simulink model "CollaborativeErgonomyControl"  (R2021b)
settings: Solver=FixedStepAuto  StartTime=0.0  StopTime=Config.SIMULATION_TIME  FixedStep=Config.tStep  RelTol=1e-3
InitFcn:
  | %% initialize the simulation
  | cd(fileparts(which(bdroot)));
  | initCollaborativeErgonomyControl;
StopFcn:
  | %% stop the simulation
  | cd(fileparts(which(bdroot)));
  | stopCollaborativeErgonomyControl;
values from neighbouring files (symbols this model uses):
  ConfigRobot1 = ConfigRobot    [initCollaborativeErgonomyControl.m]
  ConfigRobot2 = ConfigRobot    [initCollaborativeErgonomyControl.m]
undefined symbols (not defined in the file or in its folder): Config, ConfigObject
libraries: RobotStateLibrary x61, WBToolboxLibrary x40, MultiBodyLibrary x4, simulink x3
(part 2 of 2)

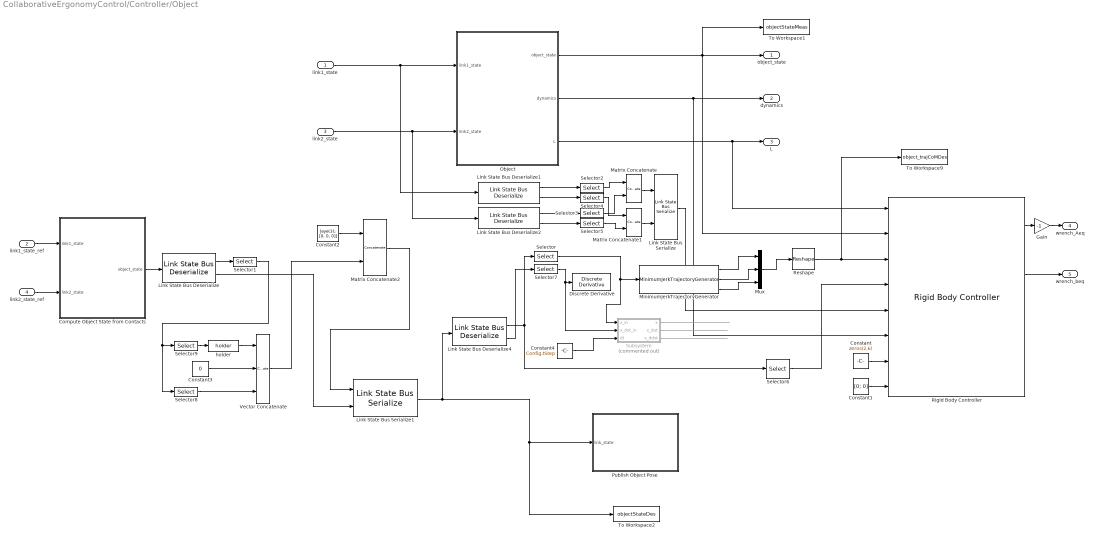
== system CollaborativeErgonomyControl/Controller/Object ==
  link1_state : Inport
  link1_state_ref : Inport  Port=2
  link2_state : Inport  Port=3
  link2_state_ref : Inport  Port=4
  Compute Object State from Contacts : Subsystem  AncestorBlock=MultiBodyLibrary/Compute Object State from Contacts
  Constant : Constant  Value=zeros(2,6)
  Constant1 : Constant  Value=[0; 0]
  Constant2 : Constant  Value=[eye(3); [0, 0, 0]]
  Constant3 : Constant  Value=0
  Constant4 : Constant  Value=Config.tStep
  Discrete Derivative : simulink/Discrete/Discrete Derivative  gainval=1.0  ICPrevScaledInput=0.0  OutMin=[]  OutMax=[]  OutDataType=fixdt(1, 16)  OutScaling=2^-10  DoSatur=off
  Gain : Gain  Gain=-1
  Link State Bus Deserialize{,1..2,4} (4 alike) : RobotStateLibrary/Link State Bus Deserialize  SystemSampleTime=-1  VariantActivationTime=update diagram  Latency=0  AutoFrameSizeCalculation=off
      settings: SourceProductName=robot-state-library
  Link State Bus Serialize : RobotStateLibrary/Link State Bus Serialize  SystemSampleTime=-1  VariantActivationTime=update diagram  Latency=0  AutoFrameSizeCalculation=off
      settings: SourceProductName=robot-state-library
  Link State Bus Serialize1 : RobotStateLibrary/Link State Bus Serialize  SystemSampleTime=-1  VariantActivationTime=update diagram  Latency=0  AutoFrameSizeCalculation=off
      settings: SourceProductName=robot-state-library
  Matrix Concatenate : Concatenate  Mode=Multidimensional array
  Matrix Concatenate1 : Concatenate  Mode=Multidimensional array
  Matrix Concatenate2 : Concatenate  Mode=Multidimensional array  ConcatenateDimension=2
  MinimumJerkTrajectoryGenerator : WBToolboxLibrary/Utilities/MinimumJerkTrajectoryGenerator  externalSettlingTime=off  settlingTime=3  sampleTime=0.01  resetOnSettlingTime=off  firstDerivatives=on  secondDerivatives=on  explicitInitialValue=off
      settings: SourceProductName=WholeBodyToolbox
  Mux : Mux  Inputs=3
  Object : Subsystem
  Publish Object Pose : Subsystem
  Reshape : Reshape  OutputDimensionality=Customize  OutputDimensions=[3,3]
  Rigid Body Controller : MultiBodyLibrary/Rigid Body Controller  GainMomentum=ConfigObject.Gains.GainMomentum  linksUseConstraintMatrix=ConfigObject.linksUseConstraintMatrix
      settings: SourceProductName=multi-body-library
  Selector : Selector  NumberOfDimensions=2  InputPortWidth=3  IndexOptions=Index vector (dialog),Index vector (dialog)  Indices=[1 2 3],4  OutputSizes=1,1
  Selector1 : Selector  NumberOfDimensions=2  InputPortWidth=3  IndexOptions=Index vector (dialog),Index vector (dialog)  Indices=[1 2 3 4],4  OutputSizes=1,1
  Selector2 : Selector  NumberOfDimensions=2  InputPortWidth=3  IndexOptions=Starting index (dialog),Index vector (dialog)  Indices=9,[1 2 3 4]  OutputSizes=8,1
  Selector3 : Selector  NumberOfDimensions=2  InputPortWidth=3  IndexOptions=Starting index (dialog),Index vector (dialog)  Indices=9,[1 2 3 4]  OutputSizes=8,1
  Selector4 : Selector  NumberOfDimensions=2  InputPortWidth=3  IndexOptions=Starting index (dialog),Index vector (dialog)  Indices=13,1  OutputSizes=12,1
  Selector5 : Selector  NumberOfDimensions=2  InputPortWidth=3  IndexOptions=Starting index (dialog),Index vector (dialog)  Indices=13,1  OutputSizes=12,1
  Selector6 : Selector  NumberOfDimensions=2  InputPortWidth=3  IndexOptions=Index vector (dialog),Index vector (dialog)  Indices=[1 2 3],[1 2 3]  OutputSizes=1,1
  Selector7 : Selector  IndexOptions=Index vector (dialog)  Indices=[1 2 3]  OutputSizes=1
  Selector8 : Selector  IndexOptions=Index vector (dialog)  Indices=[3 4]  OutputSizes=1
  Selector9 : Selector  IndexOptions=Index vector (dialog)  Indices=[1]  OutputSizes=1
  Subsystem : Subsystem  Commented=on
  To Workspace1 : ToWorkspace  VariableName=objectStateMeas  SaveFormat=Timeseries  SampleTime=-1
  To Workspace2 : ToWorkspace  VariableName=objectStateDes  SaveFormat=Timeseries  SampleTime=-1
  To Workspace9 : ToWorkspace  VariableName=object_trajCoMDes  SaveFormat=Timeseries  SampleTime=-1
  Vector Concatenate : Concatenate  NumInputs=3
  "holder " : WBToolboxLibrary/Utilities/holder 
      settings: SourceProductName=WholeBodyToolbox
  object_state : Outport
  dynamics : Outport  Port=2
  L : Outport  Port=3
  wrench_Aeq : Outport  Port=4
  wrench_beq : Outport  Port=5
  wires:
  Object/3(L) -> Rigid Body Controller/1, L/1
  link2_state_ref/1 -> Compute Object State from Contacts/2(link2_state)
  link2_state/1 -> Link State Bus Deserialize2/1, Object/2(link2_state)
  Object/1(object_state) -> To Workspace1/1, Rigid Body Controller/2, object_state/1
  Object/2(dynamics) -> Rigid Body Controller/6, dynamics/1
  link1_state_ref/1 -> Compute Object State from Contacts/1(link1_state)
  Compute Object State from Contacts/1(object_state) -> Link State Bus Deserialize/1
  Mux/1 -> Reshape/1
  Reshape/1 -> To Workspace9/1, Rigid Body Controller/3
  link1_state/1 -> Link State Bus Deserialize1/1, Object/1(link1_state)
  Link State Bus Deserialize1/1 -> Selector2/1
  Link State Bus Deserialize2/1 -> Selector3/1
  Selector2/1 -> Matrix Concatenate/1
  Selector3/1 -> Matrix Concatenate/2
  Link State Bus Deserialize1/2 -> Selector4/1
  Link State Bus Deserialize2/2 -> Selector5/1
  Selector5/1 -> Matrix Concatenate1/2
  Selector4/1 -> Matrix Concatenate1/1
  Matrix Concatenate/1 -> Link State Bus Serialize/1
  Matrix Concatenate1/1 -> Link State Bus Serialize/2
  Rigid Body Controller/1 -> Gain/1
  Rigid Body Controller/2 -> wrench_beq/1
  Gain/1 -> wrench_Aeq/1
  Constant1/1 -> Rigid Body Controller/8
  Constant/1 -> Rigid Body Controller/7
  Link State Bus Serialize/1 -> Rigid Body Controller/5
  Selector7/1 -> Subsystem/2(x_dot_in), Discrete Derivative/1
  Selector/1 -> Subsystem/1(x_in), MinimumJerkTrajectoryGenerator/1
  Selector6/1 -> Rigid Body Controller/4
  Link State Bus Deserialize/2 -> Link State Bus Serialize1/2
  Link State Bus Deserialize/1 -> Selector1/1
  Constant2/1 -> Matrix Concatenate2/1
  Matrix Concatenate2/1 -> Link State Bus Serialize1/1
  Link State Bus Serialize1/1 -> Link State Bus Deserialize4/1, To Workspace2/1, Publish Object Pose/1(link_state)
  Link State Bus Deserialize4/1 -> Selector/1, Selector6/1
  Link State Bus Deserialize4/2 -> Selector7/1
  Vector Concatenate/1 -> Matrix Concatenate2/2
  Constant3/1 -> Vector Concatenate/2
  Selector8/1 -> Vector Concatenate/3
  Selector9/1 -> "holder "/1
  "holder "/1 -> Vector Concatenate/1
  Selector1/1 -> Selector8/1, Selector9/1
  Constant4/1 -> Subsystem/3(dt)
  Subsystem/1(x) -> ?
  Subsystem/2(x_dot) -> ?
  Subsystem/3(x_ddot) -> ?
  MinimumJerkTrajectoryGenerator/1 -> Mux/1
  MinimumJerkTrajectoryGenerator/2 -> Mux/2
  MinimumJerkTrajectoryGenerator/3 -> Mux/3

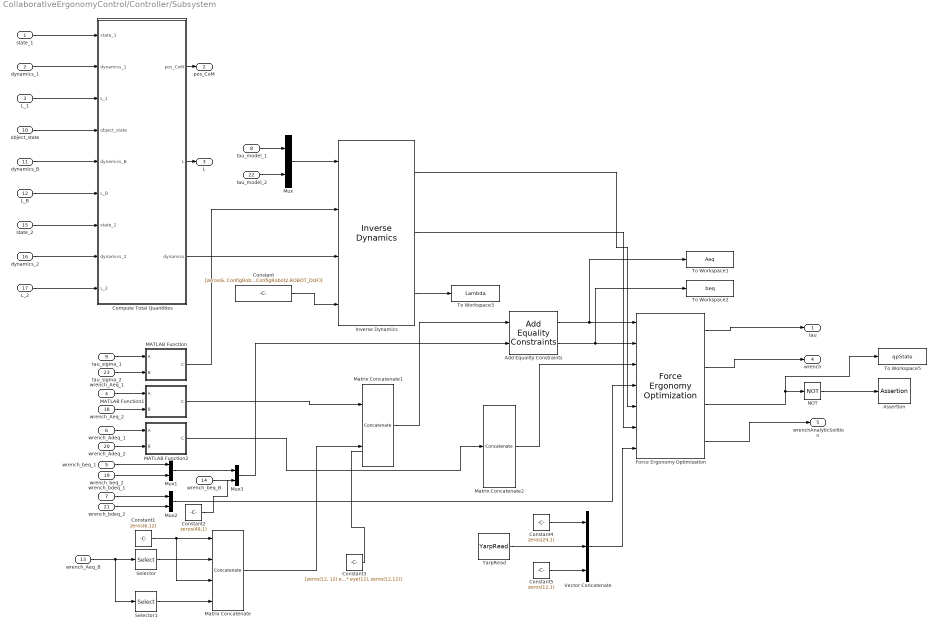
== system CollaborativeErgonomyControl/Controller/Subsystem ==
  state_1 : Inport
  dynamics_1 : Inport  Port=2
  L_1 : Inport  Port=3
  wrench_Aeq_1 : Inport  Port=4
  wrench_beq_1 : Inport  Port=5
  wrench_Adeq_1 : Inport  Port=6
  wrench_bdeq_1 : Inport  Port=7
  tau_model_1 : Inport  Port=8
  tau_sigma_1 : Inport  Port=9
  object_state : Inport  Port=10
  dynamics_B : Inport  Port=11
  L_B : Inport  Port=12
  wrench_Aeq_B : Inport  Port=13
  wrench_beq_B : Inport  Port=14
  state_2 : Inport  Port=15
  dynamics_2 : Inport  Port=16
  L_2 : Inport  Port=17
  wrench_Aeq_2 : Inport  Port=18
  wrench_beq_2 : Inport  Port=19
  wrench_Adeq_2 : Inport  Port=20
  wrench_bdeq_2 : Inport  Port=21
  tau_model_2 : Inport  Port=22
  tau_sigma_2 : Inport  Port=23
  Add Equality Constraints : RobotStateLibrary/Add Equality Constraints  Aeq_add=Config.wrench_Aeq_const  beq_add=Config.wrench_beq_const
      settings: SourceProductName=robot-state-library
  Assertion : Assertion
  Compute Total Quantities : Subsystem
  Constant : Constant  Value=[zeros(6, ConfigRobot1.ROBOT_DOF + ConfigRobot2.ROBOT_DOF); [eye(ConfigRobot1.ROBOT_DOF), zeros(ConfigRobot1.ROBOT_DOF, ConfigRobot2.ROBOT_DOF)]; zeros(6, ConfigRobot1.ROBOT_DOF + ConfigRobot2.ROBOT_DOF); [zeros(ConfigRobot2.ROBOT_DOF, ConfigRobot1.ROBOT_DOF), eye(ConfigRobot2.ROBOT_DOF)]; zeros(6, ConfigRobot1.ROBOT_DOF + ConfigRobot2.ROBOT_DOF)]
  Constant1 : Constant  Value=zeros(6,12)
  Constant2 : Constant  Value=zeros(48,1)
  Constant3 : Constant  Value=[zeros(12, 12) eye(12) zeros(12, 24); zeros(12, 24) zeros(12, 12) eye(12); 0.01 * eye(12) zeros(12,36); zeros(12,24) 0.01 * eye(12), zeros(12,12)]
  Constant4 : Constant  Value=zeros(24,1)
  Constant5 : Constant  Value=zeros(12,1)
  Force Ergonomy Optimization : RobotStateLibrary/Force Ergonomy Optimization  InvTol=Config.Reg.AInvTol  regularizationHessian=Config.Reg.Hessian  minimizationWeight=Config.Gains.tauMinimization  regularizationYDes=Config.Reg.DesWrenchReg
      settings: SourceProductName=robot-state-library
  Inverse Dynamics : RobotStateLibrary/Inverse Dynamics  Reg=Config.Reg  fixedLinkVelcityComponents=Config.fixedLinkVelcityComponents
      settings: SourceProductName=robot-state-library
  MATLAB Function : MATLAB Function  TreatAsAtomicUnit=on
  MATLAB Function1 : MATLAB Function  TreatAsAtomicUnit=on
  MATLAB Function2 : MATLAB Function  TreatAsAtomicUnit=on
  Matrix Concatenate : Concatenate  NumInputs=4  Mode=Multidimensional array  ConcatenateDimension=2
  Matrix Concatenate1 : Concatenate  Mode=Multidimensional array
  Matrix Concatenate2 : Concatenate  NumInputs=1  Mode=Multidimensional array
  Mux{,1..3} (4 alike) : Mux  Inputs=2
  NOT : Logic  Operator=NOT  IconShape=distinctive  AllPortsSameDT=off  OutDataTypeStr=boolean
  Selector : Selector  NumberOfDimensions=2  InputPortWidth=3  IndexOptions=Starting index (dialog),Starting index (dialog)  Indices=1,1  OutputSizes=6,12
  Selector1 : Selector  NumberOfDimensions=2  InputPortWidth=3  IndexOptions=Starting index (dialog),Starting index (dialog)  Indices=1,13  OutputSizes=6,12
  To Workspace1 : ToWorkspace  VariableName=Aeq  SaveFormat=Timeseries  SampleTime=-1
  To Workspace2 : ToWorkspace  VariableName=beq  SaveFormat=Timeseries  SampleTime=-1
  To Workspace3 : ToWorkspace  VariableName=Lambda  SaveFormat=Timeseries  SampleTime=-1
  To Workspace5 : ToWorkspace  VariableName=qpState  SaveFormat=Timeseries  SampleTime=-1
  Vector Concatenate : Concatenate  NumInputs=3
  YarpRead : WBToolboxLibrary/Utilities/YarpRead  portName=ConfigRobot2.Ports.WRENCH_FEET  signalSize=12  timeout=0.5  blocking=off  timestamp=off  autoconnect=on  errorOnConnection=on
      settings: SourceProductName=WholeBodyToolbox
  tau : Outport
  pos_CoM : Outport  Port=2
  L : Outport  Port=3
  wrench : Outport  Port=4
  wrenchAnalyticSolition : Outport  Port=5
  wires:
  wrench_Aeq_2/1 -> MATLAB Function1/2(B)
  Mux/1 -> Inverse Dynamics/1
  Compute Total Quantities/2(L) -> L/1
  Force Ergonomy Optimization/1 -> tau/1
  wrench_bdeq_1/1 -> Mux2/1
  Selector/1 -> Matrix Concatenate/2
  wrench_bdeq_2/1 -> Mux2/2
  state_2/1 -> Compute Total Quantities/7(state_2)
  dynamics_2/1 -> Compute Total Quantities/8(dynamics_2)
  dynamics_1/1 -> Compute Total Quantities/2(dynamics_1)
  tau_sigma_1/1 -> MATLAB Function/1(A)
  dynamics_B/1 -> Compute Total Quantities/5(dynamics_B)
  wrench_Adeq_2/1 -> MATLAB Function2/2(B)
  Compute Total Quantities/3(dynamics) -> Inverse Dynamics/3
  Mux2/1 -> Force Ergonomy Optimization/4
  object_state/1 -> Compute Total Quantities/4(object_state)
  MATLAB Function/1(C) -> Inverse Dynamics/2
  L_1/1 -> Compute Total Quantities/3(L_1)
  wrench_Aeq_1/1 -> MATLAB Function1/1(A)
  Force Ergonomy Optimization/2 -> wrench/1
  Mux3/1 -> Add Equality Constraints/2
  Constant1/1 -> Matrix Concatenate/3, Matrix Concatenate/1
  Compute Total Quantities/1(pos_CoM) -> pos_CoM/1
  wrench_Aeq_B/1 -> Selector1/1, Selector/1
  tau_model_1/1 -> Mux/1
  state_1/1 -> Compute Total Quantities/1(state_1)
  wrench_beq_2/1 -> Mux1/2
  Mux1/1 -> Mux3/1
  Matrix Concatenate1/1 -> Add Equality Constraints/1
  wrench_beq_B/1 -> Mux3/2
  Matrix Concatenate/1 -> Matrix Concatenate1/2
  MATLAB Function1/1(C) -> Matrix Concatenate1/1
  wrench_beq_1/1 -> Mux1/1
  Inverse Dynamics/1 -> Force Ergonomy Optimization/5
  tau_model_2/1 -> Mux/2
  L_B/1 -> Compute Total Quantities/6(L_B)
  Add Equality Constraints/2 -> To Workspace2/1, Force Ergonomy Optimization/2
  wrench_Adeq_1/1 -> MATLAB Function2/1(A)
  tau_sigma_2/1 -> MATLAB Function/2(B)
  L_2/1 -> Compute Total Quantities/9(L_2)
  Constant/1 -> Inverse Dynamics/4
  Inverse Dynamics/2 -> Force Ergonomy Optimization/6
  Selector1/1 -> Matrix Concatenate/4
  NOT/1 -> Assertion/1
  Force Ergonomy Optimization/3 -> To Workspace5/1, NOT/1
  Add Equality Constraints/1 -> To Workspace1/1, Force Ergonomy Optimization/1
  Force Ergonomy Optimization/4 -> wrenchAnalyticSolition/1
  Inverse Dynamics/3 -> To Workspace3/1
  MATLAB Function2/1(C) -> Matrix Concatenate2/1
  Matrix Concatenate2/1 -> Force Ergonomy Optimization/3
  Constant2/1 -> ?
  Constant3/1 -> ?
  Vector Concatenate/1 -> Force Ergonomy Optimization/7
  Constant4/1 -> Vector Concatenate/1
  YarpRead/1 -> Vector Concatenate/2
  Constant5/1 -> Vector Concatenate/3

== system CollaborativeErgonomyControl/Dump and visualize/Time Scope ==
  yarp_time : Inport
  simulink_time : Inport  Port=2
  Enable : EnablePort
  Difference : simulink/Discrete/Difference  ICPrevInput=0.0  OutMin=[]  OutMax=[]  OutDataType=fixdt(1, 16)  OutScaling=2^-10  DoSatur=off
  Difference1 : simulink/Discrete/Difference  ICPrevInput=0.0  OutMin=[]  OutMax=[]  OutDataType=fixdt(1, 16)  OutScaling=2^-10  DoSatur=off
  Minus : Sum  Inputs=-+
  Mux : Mux  Inputs=2
  Mux1 : Mux  Inputs=2
  Time Scope : Scope  NumInputPorts=2
  "holder " : WBToolboxLibrary/Utilities/holder 
      settings: SourceProductName=WholeBodyToolbox
  wires:
  yarp_time/1 -> "holder "/1, Minus/2, Difference/1  "time"
  "holder "/1 -> Minus/1
  simulink_time/1 -> Mux/2, Difference1/1  "simulink time"
  Minus/1 -> Mux/1  "yarp time"
  Mux/1 -> Time Scope/1
  Difference/1 -> Mux1/1  "yarp time step"
  Difference1/1 -> Mux1/2  "simulink time step"
  Mux1/1 -> Time Scope/2

== system CollaborativeErgonomyControl/synchronizer/GAZEBO_SYNCHRONIZER ==
  Enable : EnablePort
  Simulator Synchronizer : WBToolboxLibrary/Utilities/Simulator Synchronizer  period=Config.tStep  serverPortName='/clock/rpc'  clientPortName='/WBT_synchronizer/rpc:o'
      settings: SourceProductName=WholeBodyToolbox

== system CollaborativeErgonomyControl/synchronizer/REAL_TIME_SYNC ==
  Enable : EnablePort
  Real Time Synchronizer : WBToolboxLibrary/Utilities/Real Time Synchronizer  period=Config.tStep
      settings: SourceProductName=WholeBodyToolbox

== system CollaborativeErgonomyControl/Controller/Model 1/Initial State Holder ==
  state : Inport
  State Bus Deserializer : RobotStateLibrary/State Bus Deserializer  SystemSampleTime=-1  VariantActivationTime=update diagram  Latency=0  AutoFrameSizeCalculation=off
      settings: SourceProductName=robot-state-library
  State Bus Serializer : RobotStateLibrary/State Bus Serializer  SystemSampleTime=-1  VariantActivationTime=update diagram  Latency=0  AutoFrameSizeCalculation=off
      settings: SourceProductName=robot-state-library
  holder {,1..3} (4 alike) : WBToolboxLibrary/Utilities/holder 
      settings: SourceProductName=WholeBodyToolbox
  state0 : Outport
  wires:
  State Bus Deserializer/2 -> holder 1/1
  State Bus Deserializer/4 -> holder 3/1
  holder 1/1 -> State Bus Serializer/2
  holder 3/1 -> State Bus Serializer/4
  State Bus Deserializer/1 -> "holder "/1
  state/1 -> State Bus Deserializer/1
  holder 2/1 -> State Bus Serializer/3
  State Bus Serializer/1 -> state0/1
  "holder "/1 -> State Bus Serializer/1
  State Bus Deserializer/3 -> holder 2/1

== system CollaborativeErgonomyControl/Controller/Model 3/Initial State Holder ==
  state : Inport
  State Bus Deserializer : RobotStateLibrary/State Bus Deserializer  SystemSampleTime=-1  VariantActivationTime=update diagram  Latency=0  AutoFrameSizeCalculation=off
      settings: SourceProductName=robot-state-library
  State Bus Serializer : RobotStateLibrary/State Bus Serializer  SystemSampleTime=-1  VariantActivationTime=update diagram  Latency=0  AutoFrameSizeCalculation=off
      settings: SourceProductName=robot-state-library
  holder {,1..3} (4 alike) : WBToolboxLibrary/Utilities/holder 
      settings: SourceProductName=WholeBodyToolbox
  state0 : Outport
  wires:
  State Bus Deserializer/2 -> holder 1/1
  State Bus Deserializer/4 -> holder 3/1
  holder 1/1 -> State Bus Serializer/2
  holder 3/1 -> State Bus Serializer/4
  State Bus Deserializer/1 -> "holder "/1
  state/1 -> State Bus Deserializer/1
  holder 2/1 -> State Bus Serializer/3
  State Bus Serializer/1 -> state0/1
  "holder "/1 -> State Bus Serializer/1
  State Bus Deserializer/3 -> holder 2/1

== system CollaborativeErgonomyControl/Controller/Object/Compute Object State from Contacts ==
  link1_state : Inport
  link2_state : Inport  Port=2
  Compute Object Pose From Contacts : Subsystem
  Compute Object Velocity From Contacts : Subsystem
  Link State Bus Deserialize : RobotStateLibrary/Link State Bus Deserialize  SystemSampleTime=-1  VariantActivationTime=update diagram  Latency=0  AutoFrameSizeCalculation=off
      settings: SourceProductName=robot-state-library
  Link State Bus Deserialize1 : RobotStateLibrary/Link State Bus Deserialize  SystemSampleTime=-1  VariantActivationTime=update diagram  Latency=0  AutoFrameSizeCalculation=off
      settings: SourceProductName=robot-state-library
  Link State Bus Serialize : RobotStateLibrary/Link State Bus Serialize  SystemSampleTime=-1  VariantActivationTime=update diagram  Latency=0  AutoFrameSizeCalculation=off
      settings: SourceProductName=robot-state-library
  object_state : Outport
  wires:
  Link State Bus Serialize/1 -> object_state/1
  Compute Object Velocity From Contacts/1(v_b) -> Link State Bus Serialize/2
  link2_state/1 -> Link State Bus Deserialize1/1
  link1_state/1 -> Link State Bus Deserialize/1
  Compute Object Pose From Contacts/1(w_H_b) -> Compute Object Velocity From Contacts/5(w_H_B), Link State Bus Serialize/1
  Link State Bus Deserialize1/1 -> Compute Object Pose From Contacts/2(w_H_2), Compute Object Velocity From Contacts/4(w_H_2)
  Link State Bus Deserialize1/2 -> Compute Object Velocity From Contacts/2(v_2)
  Link State Bus Deserialize/2 -> Compute Object Velocity From Contacts/1(v_1)
  Link State Bus Deserialize/1 -> Compute Object Pose From Contacts/1(w_H_1), Compute Object Velocity From Contacts/3(w_H_1)

== system CollaborativeErgonomyControl/Controller/Object/Object ==
  link1_state : Inport
  link2_state : Inport  Port=2
  Constant : Constant  Value=ConfigObject.contacts
  Constant1 : Constant  Value=ConfigObject.MassMatrix
  Get Object State and Dynamics : MultiBodyLibrary/Get Object State and Dynamics  SystemSampleTime=-1  VariantActivationTime=update diagram  Latency=0  AutoFrameSizeCalculation=off
      settings: SourceProductName=multi-body-library
  Publish Object Pose : Subsystem
  object_state : Outport
  dynamics : Outport  Port=2
  L : Outport  Port=3
  wires:
  link1_state/1 -> Get Object State and Dynamics/1
  Get Object State and Dynamics/1 -> object_state/1, Publish Object Pose/1(link_state)
  Constant1/1 -> Get Object State and Dynamics/4
  link2_state/1 -> Get Object State and Dynamics/2
  Get Object State and Dynamics/2 -> dynamics/1
  Constant/1 -> Get Object State and Dynamics/3
  Get Object State and Dynamics/3 -> L/1

== system CollaborativeErgonomyControl/Controller/Object/Publish Object Pose ==
  link_state : Inport
  Link State Bus Deserialize : RobotStateLibrary/Link State Bus Deserialize  SystemSampleTime=-1  VariantActivationTime=update diagram  Latency=0  AutoFrameSizeCalculation=off
      settings: SourceProductName=robot-state-library
  Pose Yarp Publisher : RobotStateLibrary/Pose Yarp Publisher  portName='/collaborativeController/boxRef/basePose:o'
      settings: SourceProductName=robot-state-library
  wires:
  Link State Bus Deserialize/1 -> Pose Yarp Publisher/1
  link_state/1 -> Link State Bus Deserialize/1

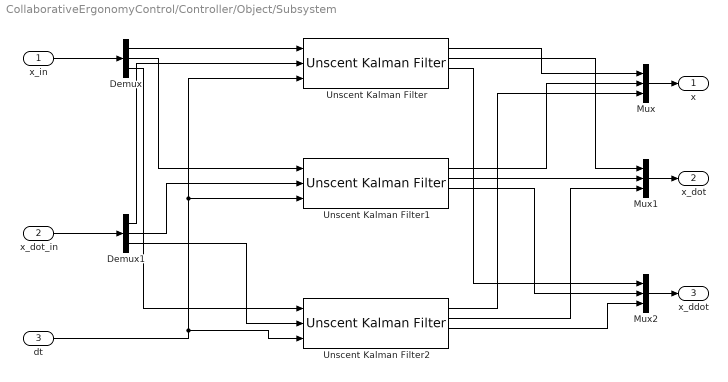
== system CollaborativeErgonomyControl/Controller/Object/Subsystem ==
  x_in : Inport
  x_dot_in : Inport  Port=2
  dt : Inport  Port=3
  Demux : Demux  Outputs=3
  Demux1 : Demux  Outputs=3
  Mux : Mux  Inputs=3
  Mux1 : Mux  Inputs=3
  Mux2 : Mux  Inputs=3
  Unscent Kalman Filter : RobotStateLibrary/Unscent Kalman Filter  SystemSampleTime=-1  VariantActivationTime=update diagram  Latency=0  AutoFrameSizeCalculation=off
      settings: SourceProductName=robot-state-library
  Unscent Kalman Filter1 : RobotStateLibrary/Unscent Kalman Filter  SystemSampleTime=-1  VariantActivationTime=update diagram  Latency=0  AutoFrameSizeCalculation=off
      settings: SourceProductName=robot-state-library
  Unscent Kalman Filter2 : RobotStateLibrary/Unscent Kalman Filter  SystemSampleTime=-1  VariantActivationTime=update diagram  Latency=0  AutoFrameSizeCalculation=off
      settings: SourceProductName=robot-state-library
  x : Outport
  x_dot : Outport  Port=2
  x_ddot : Outport  Port=3
  wires:
  x_in/1 -> Demux/1
  x_dot_in/1 -> Demux1/1
  dt/1 -> Unscent Kalman Filter2/3, Unscent Kalman Filter1/3, Unscent Kalman Filter/3
  Mux/1 -> x/1
  Mux1/1 -> x_dot/1
  Mux2/1 -> x_ddot/1
  Unscent Kalman Filter/1 -> Mux/1
  Unscent Kalman Filter1/1 -> Mux/2
  Unscent Kalman Filter2/1 -> Mux/3
  Unscent Kalman Filter/2 -> Mux1/1
  Unscent Kalman Filter1/2 -> Mux1/2
  Unscent Kalman Filter2/2 -> Mux1/3
  Unscent Kalman Filter/3 -> Mux2/1
  Unscent Kalman Filter1/3 -> Mux2/2
  Unscent Kalman Filter2/3 -> Mux2/3
  Demux/1 -> Unscent Kalman Filter/1
  Demux/2 -> Unscent Kalman Filter1/1
  Demux/3 -> Unscent Kalman Filter2/1
  Demux1/1 -> Unscent Kalman Filter/2
  Demux1/2 -> Unscent Kalman Filter1/2
  Demux1/3 -> Unscent Kalman Filter2/2

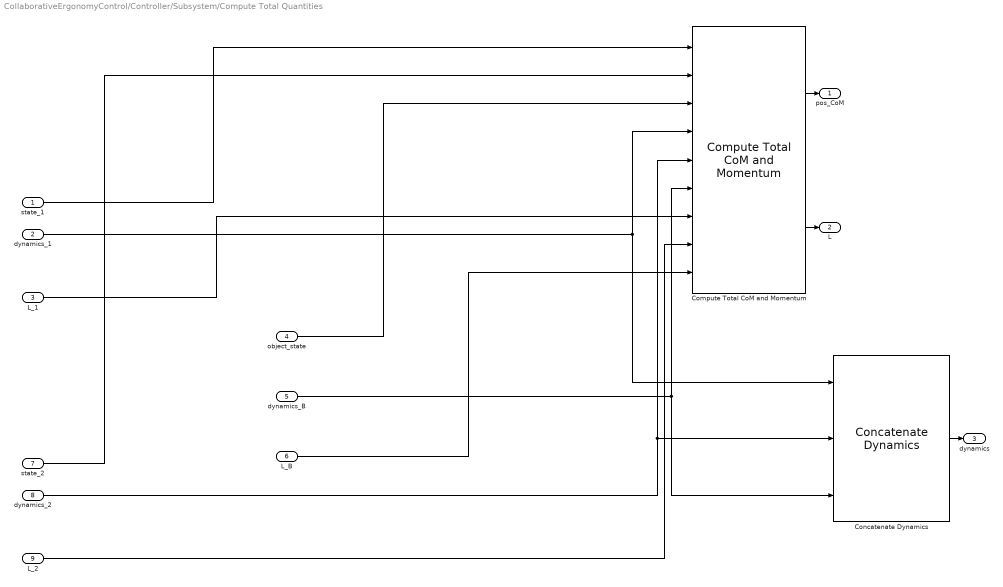
== system CollaborativeErgonomyControl/Controller/Subsystem/Compute Total Quantities ==
  state_1 : Inport
  dynamics_1 : Inport  Port=2
  L_1 : Inport  Port=3
  object_state : Inport  Port=4
  dynamics_B : Inport  Port=5
  L_B : Inport  Port=6
  state_2 : Inport  Port=7
  dynamics_2 : Inport  Port=8
  L_2 : Inport  Port=9
  Compute Total CoM and Momentum : MultiBodyLibrary/Compute Total CoM and Momentum  SystemSampleTime=-1  VariantActivationTime=update diagram  Latency=0  AutoFrameSizeCalculation=off
      settings: SourceProductName=multi-body-library
  Concatenate Dynamics : MultiBodyLibrary/Concatenate Dynamics  SystemSampleTime=-1  VariantActivationTime=update diagram  Latency=0  AutoFrameSizeCalculation=off
      settings: SourceProductName=multi-body-library
  pos_CoM : Outport
  L : Outport  Port=2
  dynamics : Outport  Port=3
  wires:
  L_2/1 -> Compute Total CoM and Momentum/8
  Compute Total CoM and Momentum/2 -> L/1
  L_B/1 -> Compute Total CoM and Momentum/9
  dynamics_2/1 -> Compute Total CoM and Momentum/5, Concatenate Dynamics/2
  Compute Total CoM and Momentum/1 -> pos_CoM/1
  dynamics_B/1 -> Compute Total CoM and Momentum/6, Concatenate Dynamics/3
  L_1/1 -> Compute Total CoM and Momentum/7
  object_state/1 -> Compute Total CoM and Momentum/3
  dynamics_1/1 -> Compute Total CoM and Momentum/4, Concatenate Dynamics/1
  Concatenate Dynamics/1 -> dynamics/1
  state_2/1 -> Compute Total CoM and Momentum/2
  state_1/1 -> Compute Total CoM and Momentum/1

== system CollaborativeErgonomyControl/Controller/Object/Compute Object State from Contacts/Compute Object Pose From Contacts ==
  w_H_1 : Inport
  w_H_2 : Inport  Port=2
  Compute Object pose from contacts : MATLAB Function  TreatAsAtomicUnit=on
  w_H_b : Outport
  wires:
  w_H_1/1 -> Compute Object pose from contacts/1(w_H_1)
  Compute Object pose from contacts/1(w_H_b) -> w_H_b/1
  w_H_2/1 -> Compute Object pose from contacts/2(w_H_2)

== system CollaborativeErgonomyControl/Controller/Object/Compute Object State from Contacts/Compute Object Velocity From Contacts ==
  v_1 : Inport
  v_2 : Inport  Port=2
  w_H_1 : Inport  Port=3
  w_H_2 : Inport  Port=4
  w_H_B : Inport  Port=5
  Compute Object velocity : MATLAB Function  TreatAsAtomicUnit=on
  v_b : Outport
  wires:
  Compute Object velocity/1(v_b) -> v_b/1
  v_2/1 -> Compute Object velocity/2(v_2)
  v_1/1 -> Compute Object velocity/1(v_1)
  w_H_B/1 -> Compute Object velocity/5(w_H_B)
  w_H_2/1 -> Compute Object velocity/4(w_H_2)
  w_H_1/1 -> Compute Object velocity/3(w_H_1)

== system CollaborativeErgonomyControl/Controller/Object/Object/Publish Object Pose ==
  link_state : Inport
  Link State Bus Deserialize : RobotStateLibrary/Link State Bus Deserialize  SystemSampleTime=-1  VariantActivationTime=update diagram  Latency=0  AutoFrameSizeCalculation=off
      settings: SourceProductName=robot-state-library
  Pose Yarp Publisher : RobotStateLibrary/Pose Yarp Publisher  portName='/collaborativeController/box/basePose:o'
      settings: SourceProductName=robot-state-library
  wires:
  Link State Bus Deserialize/1 -> Pose Yarp Publisher/1
  link_state/1 -> Link State Bus Deserialize/1

== matlab function CollaborativeErgonomyControl/Controller/Subsystem/MATLAB Function1 ==
  data: A input; C output; B input
function C = fcn(A, B)

C = blkdiag(A, B);

end

== matlab function CollaborativeErgonomyControl/Controller/Subsystem/MATLAB Function ==
  data: A input; C output; B input
function C = fcn(A, B)

C = blkdiag(A, B);

end

== matlab function CollaborativeErgonomyControl/Controller/Subsystem/MATLAB Function2 ==
  data: A input; C output; B input
function C = fcn(A, B)

C = blkdiag(A, B);

end

== matlab function CollaborativeErgonomyControl/Controller/Object/Compute Object State from Contacts/Compute Object Pose From Contacts/Compute Object pose from contacts ==
  data: w_H_1 input; w_H_b output; w_H_2 input
function w_H_b = computeObjectPoseFromContactsFCN(w_H_1, w_H_2)

w_H_b = mbl.computeObjectPoseFromContacts(w_H_1, w_H_2, true, true);

end

== matlab function CollaborativeErgonomyControl/Controller/Object/Compute Object State from Contacts/Compute Object Velocity From Contacts/Compute Object velocity ==
  data: v_1 input; v_b output; v_2 input; w_H_1 input; w_H_2 input; w_H_B input
function v_b = computeObjectVelocityFromContactsFCN(v_1, v_2, w_H_1, w_H_2, w_H_B)

v_b = mbl.computeObjectVelocityFromContacts(v_1, v_2, w_H_1, w_H_2, w_H_B);

end
